simulink model "IDM_simulation"  (R2017b)
settings: Solver=FixedStepAuto  StartTime=0.0  StopTime=inf  FixedStep=0.00005  RelTol=1e-3
values from neighbouring files (symbols this model uses):
  a_max = 3    [IDM_parameters.m]
  b = abs(start_relative_velocity_set)    [Data_analysis_0418.m]    (also in IDM_parameters.m = 1)
  delta = 4    [IDM_parameters.m]
  s_0 = 25    [IDM_parameters.m]
  T = 1.5    [IDM_parameters.m]
  v_0 = 30    [IDM_parameters.m]
settings Model: Creator=Gyubin  LastModifiedBy=Gyubin

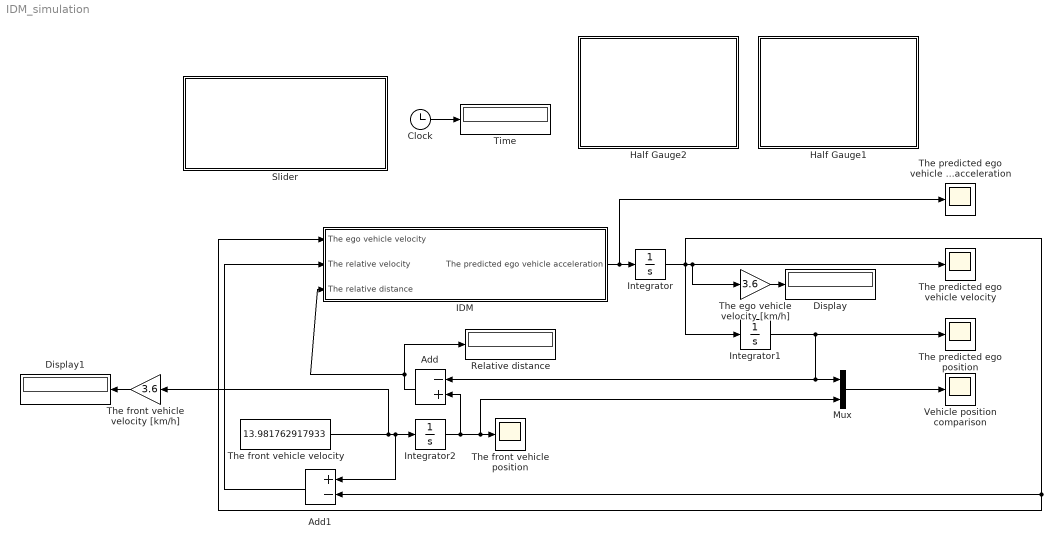
== system IDM_simulation ==
  Add : Sum  Inputs=-+
  Add1 : Sum  Inputs=+-
  Clock : Clock
  Display : Display
  Display1 : Display
  Half Gauge1 : Subsystem  DialogController=hmiCreateDDGDialog  IsWebBlock=on  mask(MWDashboardBlock){webBlockId=30af6bd7-ff31-4e87-bd5f-0def89ed546c, webBlockType=semicirculargauge, ShowInLibBrowser=on, ShowInitialText=on, HMISrcModelName=IDM_simulation}
      mask prompts: webBlockId "WebBlock Id"; webBlockType "WebBlock Type"; HMISrcModelName "Source Model"
      mask help: SimulinkHMI:dialogs:SemicircularGaugeDialogDesc
      mask Help: helpview([docroot '/mapfiles/simulink.map'], 'hmi_half_gauge')
      mask Display:
      | if strcmp(get_param(bdroot(gcb),'BlockDiagramType'), 'library')
      |     image([(matlabroot) '/toolbox/simulink/hmi/icons/SemicircularGauge.png']);
      | end
  Half Gauge2 : Subsystem  DialogController=hmiCreateDDGDialog  IsWebBlock=on  mask(MWDashboardBlock){webBlockId=b0998e06-37e1-4c8b-baf5-8251cef8b646, webBlockType=semicirculargauge, ShowInLibBrowser=on, ShowInitialText=on, HMISrcModelName=IDM_simulation}
      mask prompts: webBlockId "WebBlock Id"; webBlockType "WebBlock Type"; HMISrcModelName "Source Model"
      mask help: SimulinkHMI:dialogs:SemicircularGaugeDialogDesc
      mask Help: helpview([docroot '/mapfiles/simulink.map'], 'hmi_half_gauge')
      mask Display:
      | if strcmp(get_param(bdroot(gcb),'BlockDiagramType'), 'library')
      |     image([(matlabroot) '/toolbox/simulink/hmi/icons/SemicircularGauge.png']);
      | end
  IDM : Subsystem
  Integrator : Integrator  InitialCondition=15
  Integrator1 : Integrator
  Integrator2 : Integrator  InitialCondition=50
  Mux : Mux  Inputs=2
  Relative distance : Display
  Slider : Subsystem  DialogController=hmiCreateDDGDialog  IsWebBlock=on  mask(MWDashboardBlock){webBlockId=3da2b1f0-4bd1-4ba3-b004-775df1a0efb6, webBlockType=slider, ShowInLibBrowser=on, ShowInitialText=on, HMISrcModelName=IDM_simulation}
      mask prompts: webBlockId "WebBlock Id"; webBlockType "WebBlock Type"; HMISrcModelName "Source Model"
      mask help: SimulinkHMI:dialogs:SliderDialogDesc
      mask Help: helpview([docroot '/mapfiles/simulink.map'], 'hmi_slider')
      mask Display:
      | if strcmp(get_param(bdroot(gcb),'BlockDiagramType'), 'library')
      |     image([(matlabroot) '/toolbox/simulink/hmi/icons/Slider.png']);
      | end
  The ego vehicle velocity [km/h] : Gain  Gain=3.6
  The front vehicle position : Scope
  The front vehicle velocity : Constant  Value=13.981762917933
  The front vehicle velocity [km/h] : Gain  Gain=3.6
  The predicted ego position : Scope
  The predicted ego vehicle acceleration : Scope
  The predicted ego vehicle velocity : Scope
  Time : Display
  Vehicle position comparison : Scope
  wires:
  IDM/1(The predicted ego vehicle acceleration) -> The predicted ego vehicle acceleration/1, Integrator/1
  Integrator/1 -> The ego vehicle velocity [km/h]/1, The predicted ego vehicle velocity/1, Add1/2, IDM/1(The ego vehicle velocity), Integrator1/1
  Integrator1/1 -> Add/1, Mux/1, The predicted ego position/1
  The front vehicle velocity/1 -> The front vehicle velocity [km/h]/1, Add1/1, Integrator2/1
  Integrator2/1 -> Add/2, Mux/2, The front vehicle position/1
  Add/1 -> Relative distance/1, IDM/3(The relative distance)
  Add1/1 -> IDM/2(The relative velocity)
  Mux/1 -> Vehicle position comparison/1
  Clock/1 -> Time/1
  The ego vehicle velocity [km/h]/1 -> Display/1
  The front vehicle velocity [km/h]/1 -> Display1/1

== system IDM_simulation/Half Gauge1 ==

== system IDM_simulation/Half Gauge2 ==

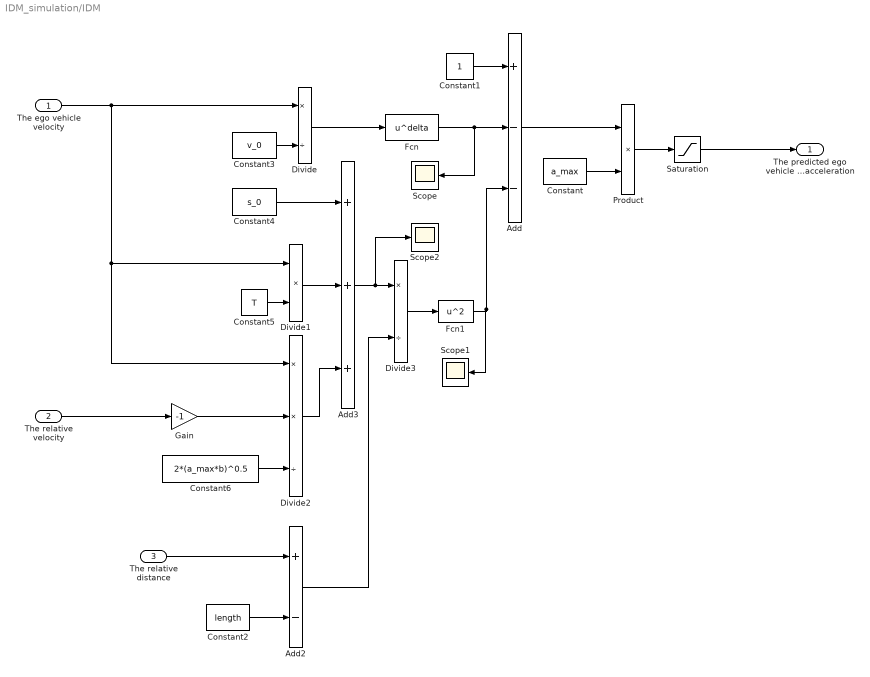
== system IDM_simulation/IDM ==
  The ego vehicle velocity : Inport
  The relative velocity : Inport  Port=2
  The relative distance : Inport  Port=3
  Add : Sum  Inputs=+--
  Add2 : Sum  Inputs=+-
  Add3 : Sum  Inputs=+++
  Constant : Constant  Value=a_max
  Constant1 : Constant
  Constant2 : Constant  Value=length
  Constant3 : Constant  Value=v_0
  Constant4 : Constant  Value=s_0
  Constant5 : Constant  Value=T
  Constant6 : Constant  Value=2*(a_max*b)^0.5
  Divide : Product  Inputs=*/
  Divide1 : Product  Inputs=**
  Divide2 : Product  Inputs=**/
  Divide3 : Product  Inputs=*/
  Fcn : Fcn  Expr=u^delta
  Fcn1 : Fcn  Expr=u^2
  Gain : Gain  Gain=-1
  Product : Product
  Saturation : Saturate  UpperLimit=19.6  LowerLimit=-19.6
  Scope : Scope
  Scope1 : Scope
  Scope2 : Scope
  The predicted ego vehicle acceleration : Outport
  wires:
  Add/1 -> Product/1
  Constant4/1 -> Add3/1
  Fcn1/1 -> Scope1/1, Add/3
  Add2/1 -> Divide3/2
  Divide3/1 -> Fcn1/1
  The relative distance/1 -> Add2/1
  Divide2/1 -> Add3/3
  Fcn/1 -> Scope/1, Add/2
  Divide/1 -> Fcn/1
  Constant1/1 -> Add/1
  Constant2/1 -> Add2/2
  Constant6/1 -> Divide2/3
  Add3/1 -> Scope2/1, Divide3/1
  Constant/1 -> Product/2
  The ego vehicle velocity/1 -> Divide2/1, Divide1/1, Divide/1
  Constant3/1 -> Divide/2
  Divide1/1 -> Add3/2
  Constant5/1 -> Divide1/2
  The relative velocity/1 -> Gain/1
  Gain/1 -> Divide2/2
  Saturation/1 -> The predicted ego vehicle acceleration/1
  Product/1 -> Saturation/1

== system IDM_simulation/Slider ==
